simulink model "Prueba_diesel"  (R2018a)
settings: Solver=ode4  StartTime=0.0  StopTime=1000  FixedStep=1e-4  RelTol=1e-3
InitFcn:
  | SimulinkInit
undefined symbols (not defined in the file): J, K1, K2, K3, P, Tao1, Tao2
libraries: simulink x1
settings Model: Creator=carma  LastModifiedBy=AndrewB
settings OptimizationCC: DefaultParameterBehavior=Inlined  EnhancedBackFolding=on  PassReuseOutputArgsAs=Individual arguments  OptimizeBlockOrder=speed  DifferentSizesBufferReuse=on  OptimizationCustomize=off
settings DebuggingCC: ParameterTunabilityLossMsg=error
settings SFSimCC: MATLABDynamicMemAlloc=off
settings RTWCC: SystemTargetFile=ert.tlc  TemplateMakefile=ert_default_tmf  GenerateReport=on  IncludeHyperlinkInReport=on  LaunchReport=on  GenerateTraceInfo=on  GenerateTraceReport=on  GenerateTraceReportSl=on  GenerateTraceReportSf=on  GenerateTraceReportEml=on
settings CodeAppCC: ForceParamTrailComments=on  IgnoreCustomStorageClasses=off  OperatorAnnotations=on  SimulinkDataObjDesc=on  SFDataObjDesc=on  InsertBlockDesc=on
settings ERTTargetCC: TargetLangStandard=C99 (ISO)  GenerateSampleERTMain=on  SupportContinuousTime=on  InlinedParameterPlacement=NonHierarchical  ERTCustomFileTemplate=example_file_process.tlc

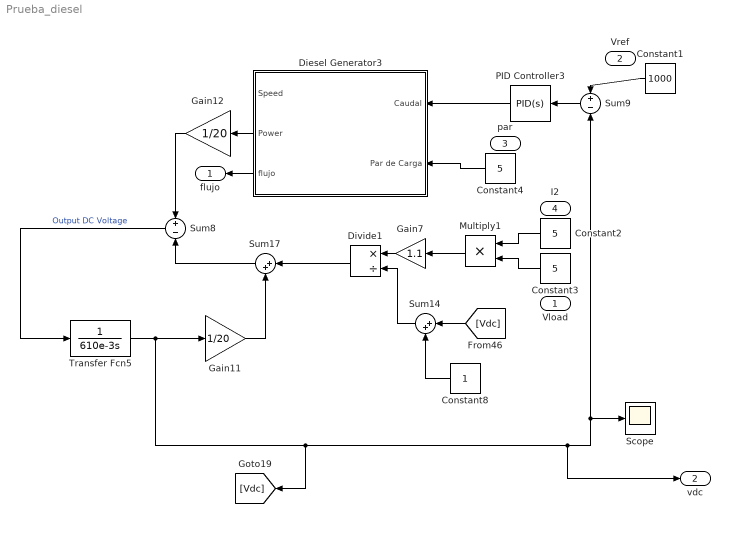
== system Prueba_diesel ==
  Vload : Inport
  Vref : Inport  Port=2
  par : Inport  Port=3
  I2 : Inport  Port=4
  Constant1 : Constant  Value=1000
  Constant2 : Constant  Value=5
  Constant3 : Constant  Value=5
  Constant4 : Constant  Value=5
  Constant8 : Constant
  Diesel Generator3 : Subsystem
  Divide1 : Product  Inputs=*/
  Gain11 : Gain  Gain=1/20
  Gain12 : Gain  Gain=1/20
  Gain7 : Gain  Gain=1.1
  Multiply1 : Product
  PID Controller3 : simulink/Continuous/PID Controller  Controller=PID  TimeDomain=Continuous-time  SampleTime=-1  IntegratorMethod=Forward Euler  FilterMethod=Forward Euler  Form=Parallel  UseFilter=on  ControllerParametersSource=internal  P=0.000853612192208084  I=3.94394231511782e-05  D=0.00224356290205903  N=0.155980576752107  InitialConditionSource=internal  InitialConditionForIntegrator=0  InitialConditionForFilter=0  ExternalReset=none  LimitOutput=off  UpperSaturationLimit=inf  LowerSaturationLimit=-inf  LinearizeAsGain=on  AntiWindupMode=none  Kb=1  TrackingMode=off  Kt=1  PParamMin=[]  PParamMax=[]  IParamMin=[]  IParamMax=[]  DParamMin=[]  DParamMax=[]  NParamMin=[]  NParamMax=[]  KbParamMin=[]  KbParamMax=[]  KtParamMin=[]  KtParamMax=[]  POutMin=[]  POutMax=[]  IOutMin=[]  IOutMax=[]  DOutMin=[]  DOutMax=[]  NOutMin=[]  NOutMax=[]  KbOutMin=[]  KbOutMax=[]  KtOutMin=[]  KtOutMax=[]  IntegratorOutMin=[]  IntegratorOutMax=[]  FilterOutMin=[]  FilterOutMax=[]  SumOutMin=[]  SumOutMax=[]  SumI1OutMin=[]  SumI1OutMax=[]  SumI2OutMin=[]  SumI2OutMax=[]  SumI3OutMin=[]  SumI3OutMax=[]  SumDOutMin=[]  SumDOutMax=[]  SaturationOutMin=[]  SaturationOutMax=[]  IntegratorContinuousStateAttributes=''  IntegratorStateMustResolveToSignalObject=off  IntegratorRTWStateStorageClass=Auto  FilterContinuousStateAttributes=''  FilterStateMustResolveToSignalObject=off  FilterRTWStateStorageClass=Auto  DifferentiatorICPrevScaledInput=0  DifferentiatorOutMin=[]  DifferentiatorOutMax=[]  InitialConditionSetting=State (most efficient)  FilterDiffOutCoefMin=[]  FilterDiffOutCoefMax=[]  SumDenOutMin=[]  SumDenOutMax=[]  SumNumOutMin=[]  SumNumOutMax=[]  ReciprocalOutMin=[]  ReciprocalOutMax=[]  DivideOutMin=[]  DivideOutMax=[]  TunerSelectOption=Transfer Function Based (PID Tuner App)
  Scope : Scope
  Sum14 : Sum  Inputs=|++
  Sum17 : Sum  Inputs=|++
  Sum8 : Sum  Inputs=+-
  Sum9 : Sum  Inputs=+-
  Transfer Fcn5 : TransferFcn  Denominator=[610e-3 0]
  flujo : Outport
  vdc : Outport  Port=2
  wires:
  PID Controller3/1 -> Diesel Generator3/1(Caudal)
  [Vdc] -> Sum14/1
  Sum8/1 -> Transfer Fcn5/1  "Output DC Voltage"
  Divide1/1 -> Sum17/1
  Transfer Fcn5/1 -> [Vdc], vdc/1, Scope/1, Sum9/2, Gain11/1
  Sum9/1 -> PID Controller3/1
  Gain12/1 -> Sum8/1
  Constant8/1 -> Sum14/2
  Sum14/1 -> Divide1/2
  Gain11/1 -> Sum17/2
  Multiply1/1 -> Gain7/1
  Diesel Generator3/3(flujo) -> flujo/1
  Diesel Generator3/2(Power) -> Gain12/1
  Sum17/1 -> Sum8/2
  Gain7/1 -> Divide1/1
  Constant1/1 -> Sum9/1
  Constant3/1 -> Multiply1/2
  Constant2/1 -> Multiply1/1
  Constant4/1 -> Diesel Generator3/2(Par de Carga)

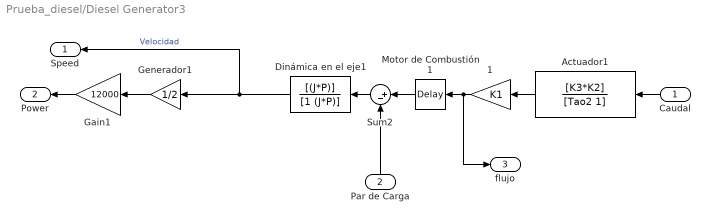
== system Prueba_diesel/Diesel Generator3 ==
  Caudal : Inport
  Par de Carga : Inport  Port=2
  " 1" : Gain  Gain=K1
  " Generador1" : Gain  Gain=1/2
  Actuador1 : TransferFcn  Numerator=[K3*K2]  Denominator=[Tao2 1]
  Dinámica en el eje1 : TransferFcn  Numerator=[(J*P)]  Denominator=[1 (J*P)]
  Gain1 : Gain  Gain=12000
  Motor de Combustión1 : TransportDelay  DelayTime=Tao1
  Sum2 : Sum  Inputs=|+-
  Speed : Outport
  Power : Outport  Port=2
  flujo : Outport  Port=3
  wires:
  " 1"/1 -> flujo/1, Motor de Combustión1/1
  " Generador1"/1 -> Gain1/1
  Motor de Combustión1/1 -> Sum2/1
  Actuador1/1 -> " 1"/1
  Dinámica en el eje1/1 -> Speed/1, " Generador1"/1  "Velocidad"
  Sum2/1 -> Dinámica en el eje1/1
  Caudal/1 -> Actuador1/1
  Par de Carga/1 -> Sum2/2
  Gain1/1 -> Power/1
